simulink model "ads5296_snap2"  (R2019a)
settings: Solver=FixedStepAuto  StartTime=0.0  StopTime=10.0  RelTol=1e-3
libraries: xbsIndex_r4 x3026, casper_library_misc x9, xps_library x1
(part 1 of 30)
settings Model: Creator=jackh  LastModifiedBy=jackh
settings DataIOCC: ReturnWorkspaceOutputs=off
settings DebuggingCC: PregeneratedLibrarySubsystemCodeDiagnostic=none  ArithmeticOperatorsInVariantConditions=warning
settings SFSimCC: SimUseLocalCustomCode=off
settings RTWCC: RTWUseLocalCustomCode=off

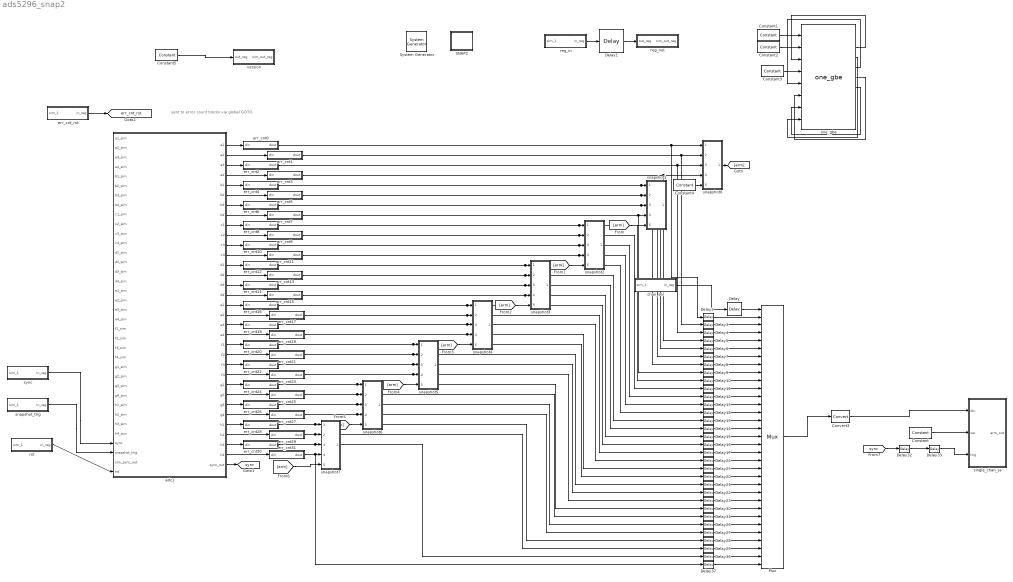
== system ads5296_snap2 ==
  note: sent to error count blocks via global GOTO.
  " System Generator" : xbsIndex_r4/ System Generator  Tag=genX  xilinxfamily=kintexu  part=xcku115  speed=-2-e  package=flvf1924  synthesis_tool=XST  clock_wrapper=Clock Enables  directory=/home/jackh/src/caltech-lwa/test_models/ads5296_snap2_clkswitch_c/sysgen  proj_type=Vivado  Synth_file=Vivado Synthesis Defaults  Impl_file=Vivado Implementation Defaults  testbench=off  simulink_period=1  sysclk_period=5  dcm_input_clock_period=10  incr_netlist=off  trim_vbits=Everywhere in SubSystem  dbl_ovrd=According to Block Masks  core_generation=According to Block Masks  run_coregen=off  deprecated_control=off  eval_field=0  block_type=sysgen
  Constant : xbsIndex_r4/Constant  const=1  gui_display_data_type=Boolean  arith_type=Boolean  n_bits=16  bin_pt=14  preci_type=Single  exp_width=8  frac_width=24  explicit_period=on  period=1  equ=P=C  opselect=C  inp2=PCIN>>17  opr=+  inp1=P  carry=CIN  dbl_ovrd=off  block_type=constant
  Constant{1..4} (4 alike) : xbsIndex_r4/Constant  const=0  gui_display_data_type=Boolean  arith_type=Boolean  n_bits=16  bin_pt=14  preci_type=Single  exp_width=8  frac_width=24  explicit_period=on  period=1  equ=P=C  opselect=C  inp2=PCIN>>17  opr=+  inp1=P  carry=CIN  dbl_ovrd=off  block_type=constant
  Constant5 : xbsIndex_r4/Constant  const=1  gui_display_data_type=Fixed-point  arith_type=Unsigned  n_bits=32  bin_pt=0  preci_type=Single  exp_width=8  frac_width=24  explicit_period=on  period=1  equ=P=C  opselect=C  inp2=PCIN>>17  opr=+  inp1=P  carry=CIN  dbl_ovrd=off  block_type=constant
  Convert3 : xbsIndex_r4/Convert  gui_display_data_type=Fixed-point  arith_type="Signed  (2's comp)"  n_bits=16  bin_pt=15  float_type=Single  exp_bits=8  fraction_bits=24  quantization=Truncate  overflow=Wrap  en=off  latency=0  pipeline=off  dbl_ovrd=off  block_type=convert
  Delay : xbsIndex_r4/Delay  rst=off  infoeditControl=Selection of Reset will increase slice count due to use of real FFs and instead of SRLs  en=off  latency=6  reg_retiming=on  dbl_ovrd=off  block_type=delay
  Delay1 : xbsIndex_r4/Delay  rst=off  infoeditControl=Selection of Reset will increase slice count due to use of real FFs and instead of SRLs  en=off  latency=1  reg_retiming=off  dbl_ovrd=off  block_type=delay
  Delay{2..32,36..37} (33 alike) : xbsIndex_r4/Delay  rst=off  infoeditControl=Selection of Reset will increase slice count due to use of real FFs and instead of SRLs  en=off  latency=2  reg_retiming=on  dbl_ovrd=off  block_type=delay
  Delay33 : xbsIndex_r4/Delay  rst=off  infoeditControl=Selection of Reset will increase slice count due to use of real FFs and instead of SRLs  en=off  latency=4  reg_retiming=on  dbl_ovrd=off  block_type=delay
  Mux : xbsIndex_r4/Mux  inputs=32  en=off  latency=4  precision=Full  arith_type=Unsigned  n_bits=16  bin_pt=14  quantization=Truncate  overflow=Wrap  dbl_ovrd=off  block_type=mux
  SNAP2 : Subsystem  Tag=xps:xsg  mask(xsg core config){hw_sys=SNAP2_v2:xcku115, clk_src=adc1_clk, clk_rate=200, use_microblaze=on, sample_period=1, synthesis_tool=XST}
      mask prompts: hw_sys "Hardware Platform"; clk_src "User IP Clock source"; clk_rate "User IP Clock Rate (MHz)"; use_microblaze "Use Microblaze controller?"; sample_period "Sample Period"; synthesis_tool "Synthesis Tool:"
      mask help:
      | The XSG Core Config block is used to configure the System Generator design
      | for the casper_xps toolflow. Settings here are used to configure the
      | Xilinx System Generator block parameters automatically, and control toolflow
      | script  execution. It needs to be at the top level of all designs being compiled
      | with the casper_xps toolflow.
      mask init:
      | xps_xsg_snap2_conf_mask;
      mask Help: eval('xlWeb([getenv(''MLIB_ROOT''), ''\doc\html\sys_xsg_core_config\sys_xsg_core_config.html''])')
      mask TypeOptions hw_sys: SNAP2_v1:xcku115 | SNAP2_v2:xcku115
      mask TypeOptions clk_src: sys_clk | clk_250MHz | adc0_clk | adc1_clk
      mask TypeOptions synthesis_tool: Leonardo Spectrum | Synplify | Synplify Pro | XST
      mask Display: fprintf(['SNAP2']);
  adc1 : Subsystem  Tag=xps:ads5296x4  mask(ADS5296x4){board_count=2, sample_rate=200, port=1, clockport=1, version=1}
      mask prompts: board_count "Number of quad-chip ADC Boards"; sample_rate "Sample Rate"; port "Which FMC port?"; clockport "Use clock from which FMC board?"; version "Which ADC board version?"
      mask help: 16-input ADC based on the TI ADS5296 chip.
      mask init:
      | % Only board_count is needed by init function
      | ads5296x4_init(gcb, ...
      |     'board_count', board_count);
      mask TypeOptions board_count: 1 | 2 | 3 | 4
  chan_sel : Subsystem  Tag=xps:sw_reg  AncestorBlock=xps_library/Memory/software_register  mask(swreg){io_dir=From Processor, io_delay=0, init_val=0, sample_period=1, names=reg, bitwidths=5, bin_pts=0, arith_types=0, sim_port=on, show_format=on}
      mask prompts: io_dir "I/O direction"; io_delay "I/O delay"; init_val "Initial Value"; sample_period "Sample period"; names "Bitfield names [msb...lsb]"; bitwidths "Bitfield widths"; bin_pts "Bitfield binary pts"; arith_types "Bitfield types, ufix=0, fix=1, bool=2"; sim_port "Provide sim input/output?"; show_format "Print format string?"
      mask help: A 32-bit software-accessible register. Can be divided into bitfields of varying widths and types using the fields in the block mask.
      mask init:
      | swreg_init(gcb)
      settings: AttributesFormatString=1input:uf5.0 = 5 bits
      mask TypeOptions io_dir: To Processor | From Processor
      mask Callback io_dir:
      | mask_enables = get_param(gcb, 'MaskEnables');
      | mask_names = get_param(gcb, 'MaskNames');
      | if strcmp(get_param(gcb, 'io_dir'), 'To Processor'),
      |     mask_enables{ismember(mask_names, 'sample_period')} = 'off';
      | else
      |     mask_enables{ismember(mask_names, 'sample_period')} = 'on';
      | end
      | set_param(gcb, 'MaskEnables', mask_enables);
      mask DialogControl ParameterTabVar0 Prompt: Setup
  err_cnt0 : Subsystem  VariantControl=Variant1
  err_cnt1 : Subsystem  VariantControl=Variant1
  err_cnt10 : Subsystem  VariantControl=Variant1
  err_cnt11 : Subsystem  VariantControl=Variant1
  err_cnt12 : Subsystem  VariantControl=Variant1
  err_cnt13 : Subsystem  VariantControl=Variant1
  err_cnt14 : Subsystem  VariantControl=Variant1
  err_cnt15 : Subsystem  VariantControl=Variant1
  err_cnt16 : Subsystem  VariantControl=Variant1
  err_cnt17 : Subsystem  VariantControl=Variant1
  err_cnt18 : Subsystem  VariantControl=Variant1
  err_cnt19 : Subsystem  VariantControl=Variant1
  err_cnt2 : Subsystem  VariantControl=Variant1
  err_cnt20 : Subsystem  VariantControl=Variant1
  err_cnt21 : Subsystem  VariantControl=Variant1
  err_cnt22 : Subsystem  VariantControl=Variant1
  err_cnt23 : Subsystem  VariantControl=Variant1
  err_cnt24 : Subsystem  VariantControl=Variant1
  err_cnt25 : Subsystem  VariantControl=Variant1
  err_cnt26 : Subsystem  VariantControl=Variant1
  err_cnt27 : Subsystem  VariantControl=Variant1
  err_cnt28 : Subsystem  VariantControl=Variant1
  err_cnt29 : Subsystem  VariantControl=Variant1
  err_cnt3 : Subsystem  VariantControl=Variant1
  err_cnt30 : Subsystem  VariantControl=Variant1
  err_cnt31 : Subsystem  VariantControl=Variant1
  err_cnt4 : Subsystem  VariantControl=Variant1
  err_cnt5 : Subsystem  VariantControl=Variant1
  err_cnt6 : Subsystem  VariantControl=Variant1
  err_cnt7 : Subsystem  VariantControl=Variant1
  err_cnt8 : Subsystem  VariantControl=Variant1
  err_cnt9 : Subsystem  VariantControl=Variant1
  err_cnt_rst : Subsystem  Tag=xps:sw_reg  AncestorBlock=xps_library/Memory/software_register  mask(swreg){io_dir=From Processor, io_delay=0, init_val=0, sample_period=1, names=reg, bitwidths=1, bin_pts=0, arith_types=2, sim_port=on, show_format=on}
      mask prompts: io_dir "I/O direction"; io_delay "I/O delay"; init_val "Initial Value"; sample_period "Sample period"; names "Bitfield names [msb...lsb]"; bitwidths "Bitfield widths"; bin_pts "Bitfield binary pts"; arith_types "Bitfield types, ufix=0, fix=1, bool=2"; sim_port "Provide sim input/output?"; show_format "Print format string?"
      mask help: A 32-bit software-accessible register. Can be divided into bitfields of varying widths and types using the fields in the block mask.
      mask init:
      | swreg_init(gcb)
      settings: AttributesFormatString=1input:b = 1 bits
      mask TypeOptions io_dir: To Processor | From Processor
      mask Callback io_dir:
      | mask_enables = get_param(gcb, 'MaskEnables');
      | mask_names = get_param(gcb, 'MaskNames');
      | if strcmp(get_param(gcb, 'io_dir'), 'To Processor'),
      |     mask_enables{ismember(mask_names, 'sample_period')} = 'off';
      | else
      |     mask_enables{ismember(mask_names, 'sample_period')} = 'on';
      | end
      | set_param(gcb, 'MaskEnables', mask_enables);
      mask DialogControl ParameterTabVar0 Prompt: Setup
  one_gbe : xps_library/IO/one_gbe  Tag=xps:onegbe  local_en=on  dis_cpu_rx=off  dis_cpu_tx=off  cpu_promiscuous=on  local_mac=hex2dec('123456789abc')  local_ip=hex2dec('c0a8290a')  local_port=4321  local_gateway=1
      settings: SourceProductName=CASPER XPS Blockset
  reg_in : Subsystem  Tag=xps:sw_reg  AncestorBlock=xps_library/Memory/software_register  mask(swreg){io_dir=From Processor, io_delay=0, init_val=0, sample_period=1, names=reg, bitwidths=10, bin_pts=9, arith_types=1, sim_port=on, show_format=on}
      mask prompts: io_dir "I/O direction"; io_delay "I/O delay"; init_val "Initial Value"; sample_period "Sample period"; names "Bitfield names [msb...lsb]"; bitwidths "Bitfield widths"; bin_pts "Bitfield binary pts"; arith_types "Bitfield types, ufix=0, fix=1, bool=2"; sim_port "Provide sim input/output?"; show_format "Print format string?"
      mask help: A 32-bit software-accessible register. Can be divided into bitfields of varying widths and types using the fields in the block mask.
      mask init:
      | swreg_init(gcb)
      settings: AttributesFormatString=1input:f10.9 = 10 bits
      mask TypeOptions io_dir: To Processor | From Processor
      mask Callback io_dir:
      | mask_enables = get_param(gcb, 'MaskEnables');
      | mask_names = get_param(gcb, 'MaskNames');
      | if strcmp(get_param(gcb, 'io_dir'), 'To Processor'),
      |     mask_enables{ismember(mask_names, 'sample_period')} = 'off';
      | else
      |     mask_enables{ismember(mask_names, 'sample_period')} = 'on';
      | end
      | set_param(gcb, 'MaskEnables', mask_enables);
      mask DialogControl ParameterTabVar0 Prompt: Setup
  reg_out : Subsystem  Tag=xps:sw_reg  AncestorBlock=xps_library/Memory/software_register  mask(swreg){io_dir=To Processor, io_delay=0, init_val=0, sample_period=1, names=reg, bitwidths=10, bin_pts=9, arith_types=1, sim_port=on, show_format=on}
      mask prompts: io_dir "I/O direction"; io_delay "I/O delay"; init_val "Initial Value"; sample_period "Sample period"; names "Bitfield names [msb...lsb]"; bitwidths "Bitfield widths"; bin_pts "Bitfield binary pts"; arith_types "Bitfield types, ufix=0, fix=1, bool=2"; sim_port "Provide sim input/output?"; show_format "Print format string?"
      mask help: A 32-bit software-accessible register. Can be divided into bitfields of varying widths and types using the fields in the block mask.
      mask init:
      | swreg_init(gcb)
      settings: AttributesFormatString=1output:f10.9 = 10 bits
      mask TypeOptions io_dir: To Processor | From Processor
      mask Callback io_dir:
      | mask_enables = get_param(gcb, 'MaskEnables');
      | mask_names = get_param(gcb, 'MaskNames');
      | if strcmp(get_param(gcb, 'io_dir'), 'To Processor'),
      |     mask_enables{ismember(mask_names, 'sample_period')} = 'off';
      | else
      |     mask_enables{ismember(mask_names, 'sample_period')} = 'on';
      | end
      | set_param(gcb, 'MaskEnables', mask_enables);
      mask DialogControl ParameterTabVar0 Prompt: Setup
  rst : Subsystem  Tag=xps:sw_reg  AncestorBlock=xps_library/Memory/software_register  mask(swreg){io_dir=From Processor, io_delay=0, init_val=0, sample_period=1, names=reg, bitwidths=1, bin_pts=0, arith_types=2, sim_port=on, show_format=on}
      mask prompts: io_dir "I/O direction"; io_delay "I/O delay"; init_val "Initial Value"; sample_period "Sample period"; names "Bitfield names [msb...lsb]"; bitwidths "Bitfield widths"; bin_pts "Bitfield binary pts"; arith_types "Bitfield types, ufix=0, fix=1, bool=2"; sim_port "Provide sim input/output?"; show_format "Print format string?"
      mask help: A 32-bit software-accessible register. Can be divided into bitfields of varying widths and types using the fields in the block mask.
      mask init:
      | swreg_init(gcb)
      settings: AttributesFormatString=1input:b = 1 bits
      mask TypeOptions io_dir: To Processor | From Processor
      mask Callback io_dir:
      | mask_enables = get_param(gcb, 'MaskEnables');
      | mask_names = get_param(gcb, 'MaskNames');
      | if strcmp(get_param(gcb, 'io_dir'), 'To Processor'),
      |     mask_enables{ismember(mask_names, 'sample_period')} = 'off';
      | else
      |     mask_enables{ismember(mask_names, 'sample_period')} = 'on';
      | end
      | set_param(gcb, 'MaskEnables', mask_enables);
      mask DialogControl ParameterTabVar0 Prompt: Setup
  single_chan_ss : Subsystem  Tag=casper:snapshot  AncestorBlock=casper_library_scopes/snapshot  mask(snapshot){storage=bram, dram_dimm=2, dram_clock=250, nsamples=16, data_width=16, offset=off, circap=off, value=off, ext_arm=off, ext_circ=off, provide_outputs=on, use_dsp48=off}
      mask prompts: storage "Storage medium"; dram_dimm "DRAM dimm"; dram_clock "DRAM clock rate"; nsamples "Number of Samples (2^?)"; data_width "Data width"; offset "Start delay support"; circap "Circular capture support"; value "Extra value capture support"; ext_arm "External arm support"; ext_circ "External circular capture support"; provide_outputs "Provide outputs"; use_dsp48 "Use DSP48s to implement counters"
      mask help:
      | Standard snap block, but with the following optional extras;
      |  1) Optionally delay the fabric trigger by a user-specified number of valids.
      |  2) Capture continuously after a trigger until a stop pulse is received. Data is captured into BRAM continuously, with old data being overwritten until a stop command is received. Then stop capturing when memory is filled. This enables you to get some data before and some data after the stop pulse. Use the 'tr_en_cnt' register to determine where you are in your vector. 'Addr' register's MSb now indicates 'busy capturing'.
      |  3) Optionally capture a value on an input port to a register at the same time as the first data sample.
      |  4) Implement counters using DSP48Es to save resources.
      mask init:
      | snapshot_init(gcb, ...
      |     'storage', storage, ...
      |     'dram_dimm', dram_dimm, ...
      |     'dram_clock', dram_clock, ...
      |     'nsamples', nsamples, ...
      |     'data_width', data_width, ...
      |     'offset', offset, ...
      |     'circap', circap, ...
      |     'value', value, ...
      |     'ext_arm', ext_arm, ...
      |     'ext_circ', ext_circ, ...
      |     'provide_outputs', 'off', ...
      |     'use_dsp48', use_dsp48);
      settings: AttributesFormatString=|
      | 16 wide, 65536 deep
      | debugID: 35264124
      mask TypeOptions storage: bram | dram
      mask Callback storage: snapshot_callback();
      mask TypeOptions dram_dimm: 1 | 2 | 3 | 4
      mask TypeOptions dram_clock: 200 | 250 | 266 | 300 | 333
      mask TypeOptions data_width: 8 | 16 | 32 | 64 | 128
  snapshot0 : Subsystem
  snapshot1 : Subsystem
  snapshot2 : Subsystem
  snapshot3 : Subsystem
  snapshot4 : Subsystem
  snapshot5 : Subsystem
  snapshot6 : Subsystem
  snapshot7 : Subsystem
  snapshot_trig : Subsystem  Tag=xps:sw_reg  AncestorBlock=xps_library/Memory/software_register  mask(swreg){io_dir=From Processor, io_delay=0, init_val=0, sample_period=1, names=reg, bitwidths=1, bin_pts=0, arith_types=2, sim_port=on, show_format=on}
      mask prompts: io_dir "I/O direction"; io_delay "I/O delay"; init_val "Initial Value"; sample_period "Sample period"; names "Bitfield names [msb...lsb]"; bitwidths "Bitfield widths"; bin_pts "Bitfield binary pts"; arith_types "Bitfield types, ufix=0, fix=1, bool=2"; sim_port "Provide sim input/output?"; show_format "Print format string?"
      mask help: A 32-bit software-accessible register. Can be divided into bitfields of varying widths and types using the fields in the block mask.
      mask init:
      | swreg_init(gcb)
      settings: AttributesFormatString=1input:b = 1 bits
      mask TypeOptions io_dir: To Processor | From Processor
      mask Callback io_dir:
      | mask_enables = get_param(gcb, 'MaskEnables');
      | mask_names = get_param(gcb, 'MaskNames');
      | if strcmp(get_param(gcb, 'io_dir'), 'To Processor'),
      |     mask_enables{ismember(mask_names, 'sample_period')} = 'off';
      | else
      |     mask_enables{ismember(mask_names, 'sample_period')} = 'on';
      | end
      | set_param(gcb, 'MaskEnables', mask_enables);
      mask DialogControl ParameterTabVar0 Prompt: Setup
  sync : Subsystem  Tag=xps:sw_reg  AncestorBlock=xps_library/Memory/software_register  mask(swreg){io_dir=From Processor, io_delay=0, init_val=0, sample_period=1, names=reg, bitwidths=1, bin_pts=0, arith_types=2, sim_port=on, show_format=on}
      mask prompts: io_dir "I/O direction"; io_delay "I/O delay"; init_val "Initial Value"; sample_period "Sample period"; names "Bitfield names [msb...lsb]"; bitwidths "Bitfield widths"; bin_pts "Bitfield binary pts"; arith_types "Bitfield types, ufix=0, fix=1, bool=2"; sim_port "Provide sim input/output?"; show_format "Print format string?"
      mask help: A 32-bit software-accessible register. Can be divided into bitfields of varying widths and types using the fields in the block mask.
      mask init:
      | swreg_init(gcb)
      settings: AttributesFormatString=1input:b = 1 bits
      mask TypeOptions io_dir: To Processor | From Processor
      mask Callback io_dir:
      | mask_enables = get_param(gcb, 'MaskEnables');
      | mask_names = get_param(gcb, 'MaskNames');
      | if strcmp(get_param(gcb, 'io_dir'), 'To Processor'),
      |     mask_enables{ismember(mask_names, 'sample_period')} = 'off';
      | else
      |     mask_enables{ismember(mask_names, 'sample_period')} = 'on';
      | end
      | set_param(gcb, 'MaskEnables', mask_enables);
      mask DialogControl ParameterTabVar0 Prompt: Setup
  version : Subsystem  Tag=xps:sw_reg  AncestorBlock=xps_library/Memory/software_register  mask(swreg){io_dir=To Processor, io_delay=0, init_val=0, sample_period=1, names=reg, bitwidths=32, bin_pts=0, arith_types=0, sim_port=on, show_format=on}
      mask prompts: io_dir "I/O direction"; io_delay "I/O delay"; init_val "Initial Value"; sample_period "Sample period"; names "Bitfield names [msb...lsb]"; bitwidths "Bitfield widths"; bin_pts "Bitfield binary pts"; arith_types "Bitfield types, ufix=0, fix=1, bool=2"; sim_port "Provide sim input/output?"; show_format "Print format string?"
      mask help: A 32-bit software-accessible register. Can be divided into bitfields of varying widths and types using the fields in the block mask.
      mask init:
      | swreg_init(gcb)
      settings: AttributesFormatString=1output:uf32.0 = 32 bits
      mask TypeOptions io_dir: To Processor | From Processor
      mask Callback io_dir:
      | mask_enables = get_param(gcb, 'MaskEnables');
      | mask_names = get_param(gcb, 'MaskNames');
      | if strcmp(get_param(gcb, 'io_dir'), 'To Processor'),
      |     mask_enables{ismember(mask_names, 'sample_period')} = 'off';
      | else
      |     mask_enables{ismember(mask_names, 'sample_period')} = 'on';
      | end
      | set_param(gcb, 'MaskEnables', mask_enables);
      mask DialogControl ParameterTabVar0 Prompt: Setup
  tag scope: err_cnt_rst=global, sync=global
  wires:
  reg_in/1(in_reg) -> Delay1/1
  Delay1/1 -> reg_out/1(out_reg)
  sync/1(in_reg) -> adc1/33(sync)
  rst/1(in_reg) -> adc1/36(rst)
  adc1/4(a4) -> err_cnt3/1(din)
  adc1/3(a3) -> err_cnt2/1(din)
  adc1/2(a2) -> err_cnt1/1(din)
  Constant1/1 -> one_gbe/1
  Constant2/1 -> one_gbe/2
  one_gbe/3 -> one_gbe/3
  Constant3/1 -> one_gbe/4
  one_gbe/5 -> one_gbe/5
  one_gbe/6 -> one_gbe/6
  one_gbe/7 -> one_gbe/7
  one_gbe/4 -> one_gbe/8
  Constant4/1 -> snapshot0/5(arm_in)
  [arm] -> snapshot1/5(arm_in)
  snapshot0/1(arm) -> [arm]
  adc1/5(b1) -> err_cnt4/1(din)
  adc1/6(b2) -> err_cnt5/1(din)
  adc1/7(b3) -> err_cnt6/1(din)
  adc1/8(b4) -> err_cnt7/1(din)
  adc1/12(c4) -> err_cnt11/1(din)
  adc1/11(c3) -> err_cnt10/1(din)
  adc1/10(c2) -> err_cnt9/1(din)
  adc1/9(c1) -> err_cnt8/1(din)
  [arm] -> snapshot2/5(arm_in)
  [arm] -> snapshot3/5(arm_in)
  adc1/13(d1) -> err_cnt12/1(din)
  adc1/14(d2) -> err_cnt13/1(din)
  adc1/15(d3) -> err_cnt14/1(din)
  adc1/16(d4) -> err_cnt15/1(din)
  [arm] -> snapshot4/5(arm_in)
  adc1/17(e1) -> err_cnt16/1(din)
  adc1/18(e2) -> err_cnt17/1(din)
  [arm] -> snapshot5/5(arm_in)
  [arm] -> snapshot6/5(arm_in)
  adc1/21(f1) -> err_cnt20/1(din)
  adc1/23(f3) -> err_cnt22/1(din)
  adc1/25(g1) -> err_cnt24/1(din)
  adc1/27(g3) -> err_cnt26/1(din)
  [arm] -> snapshot7/5(arm_in)
  adc1/29(h1) -> err_cnt28/1(din)
  adc1/30(h2) -> err_cnt29/1(din)
  adc1/31(h3) -> err_cnt30/1(din)
  adc1/32(h4) -> err_cnt31/1(din)
  adc1/33(sync_out) -> [sync]
  chan_sel/1(in_reg) -> Delay/1
  Delay/1 -> Mux/1
  Delay2/1 -> Mux/2
  Delay3/1 -> Mux/3
  Delay4/1 -> Mux/4
  Delay5/1 -> Mux/5
  Delay6/1 -> Mux/6
  Delay7/1 -> Mux/7
  Delay8/1 -> Mux/8
  Delay13/1 -> Mux/13
  Delay9/1 -> Mux/9
  Delay12/1 -> Mux/12
  Delay10/1 -> Mux/10
  Delay11/1 -> Mux/11
  Delay19/1 -> Mux/15
  Delay17/1 -> Mux/19
  Delay14/1 -> Mux/16
  Delay16/1 -> Mux/18
  Delay18/1 -> Mux/14
  Delay15/1 -> Mux/17
  Delay20/1 -> Mux/22
  Delay23/1 -> Mux/25
  Delay24/1 -> Mux/20
  Delay25/1 -> Mux/21
  Delay21/1 -> Mux/23
  Delay22/1 -> Mux/24
  Delay27/1 -> Mux/29
  Delay30/1 -> Mux/26
  Delay29/1 -> Mux/31
  Delay31/1 -> Mux/27
  Delay26/1 -> Mux/28
  Delay28/1 -> Mux/30
  Delay37/1 -> Mux/33
  Delay36/1 -> Mux/32
  [sync] -> Delay32/1
  Constant/1 -> single_chan_ss/2(we)
  Convert3/1 -> single_chan_ss/1(din)
  Mux/1 -> Convert3/1
  Delay32/1 -> Delay33/1
  Delay33/1 -> single_chan_ss/3(trig)
  err_cnt_rst/1(in_reg) -> [err_cnt_rst]
  err_cnt1/1(dout) -> snapshot0/2(din1), Delay3/1
  err_cnt2/1(dout) -> Delay4/1, snapshot0/3(din2)
  err_cnt3/1(dout) -> Delay5/1, snapshot0/4(din3)
  err_cnt5/1(dout) -> snapshot1/2(din1), Delay7/1
  err_cnt7/1(dout) -> Delay9/1, snapshot1/4(din3)
  err_cnt4/1(dout) -> snapshot1/1(din0), Delay6/1
  err_cnt6/1(dout) -> snapshot1/3(din2), Delay8/1
  err_cnt13/1(dout) -> Delay19/1, snapshot3/2(din1)
  err_cnt8/1(dout) -> Delay10/1, snapshot2/1(din0)
  err_cnt9/1(dout) -> snapshot2/2(din1), Delay11/1
  err_cnt14/1(dout) -> Delay14/1, snapshot3/3(din2)
  err_cnt15/1(dout) -> snapshot3/4(din3), Delay15/1
  err_cnt10/1(dout) -> snapshot2/3(din2), Delay12/1
  err_cnt11/1(dout) -> snapshot2/4(din3), Delay13/1
  err_cnt12/1(dout) -> snapshot3/1(din0), Delay18/1
  adc1/19(e3) -> err_cnt18/1(din)
  err_cnt22/1(dout) -> snapshot5/3(din2), Delay22/1
  adc1/22(f2) -> err_cnt21/1(din)
  adc1/24(f4) -> err_cnt23/1(din)
  err_cnt16/1(dout) -> snapshot4/1(din0), Delay16/1
  err_cnt20/1(dout) -> Delay20/1, snapshot5/1(din0)
  adc1/20(e4) -> err_cnt19/1(din)
  err_cnt17/1(dout) -> snapshot4/2(din1), Delay17/1
  err_cnt26/1(dout) -> snapshot6/3(din2), Delay26/1
  adc1/28(g4) -> err_cnt27/1(din)
  err_cnt28/1(dout) -> Delay28/1, snapshot7/1(din0)
  err_cnt29/1(dout) -> snapshot7/2(din1), Delay29/1
  err_cnt30/1(dout) -> snapshot7/3(din2), Delay36/1
  err_cnt31/1(dout) -> Delay37/1, snapshot7/4(din3)
  err_cnt24/1(dout) -> Delay30/1, snapshot6/1(din0)
  adc1/26(g2) -> err_cnt25/1(din)
  err_cnt18/1(dout) -> snapshot4/3(din2), Delay24/1
  err_cnt19/1(dout) -> Delay25/1, snapshot4/4(din3)
  err_cnt21/1(dout) -> snapshot5/2(din1), Delay21/1
  err_cnt23/1(dout) -> snapshot5/4(din3), Delay23/1
  err_cnt25/1(dout) -> Delay31/1, snapshot6/2(din1)
  err_cnt27/1(dout) -> snapshot6/4(din3), Delay27/1
  adc1/1(a1) -> err_cnt0/1(din)
  err_cnt0/1(dout) -> snapshot0/1(din0), Delay2/1
  snapshot_trig/1(in_reg) -> adc1/34(snapshot_trig)
  Constant5/1 -> version/1(out_reg)

== system ads5296_snap2/SNAP2 ==

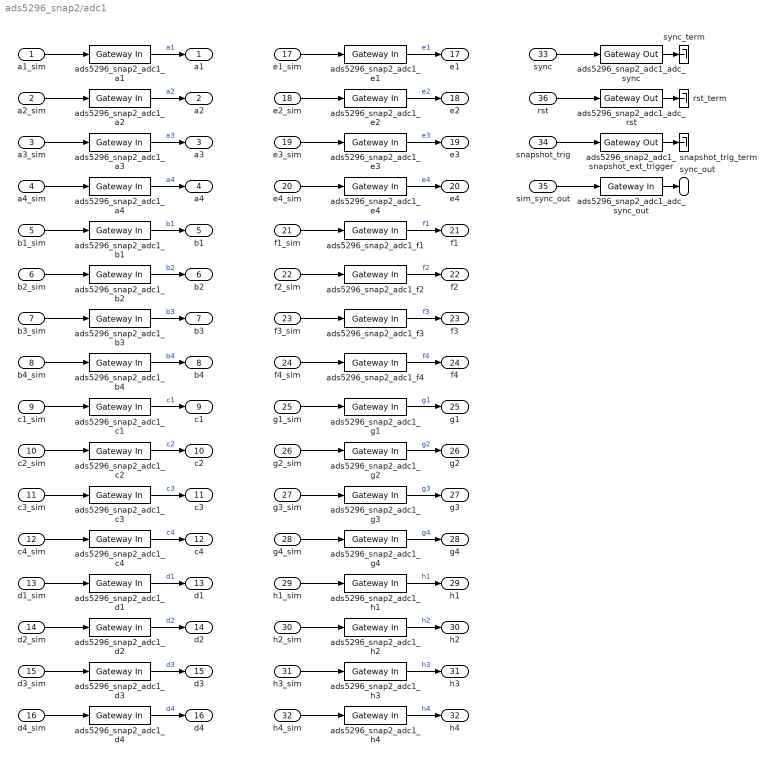
== system ads5296_snap2/adc1 ==
  a1_sim : Inport
  a2_sim : Inport  Port=2
  a3_sim : Inport  Port=3
  a4_sim : Inport  Port=4
  b1_sim : Inport  Port=5
  b2_sim : Inport  Port=6
  b3_sim : Inport  Port=7
  b4_sim : Inport  Port=8
  c1_sim : Inport  Port=9
  c2_sim : Inport  Port=10
  c3_sim : Inport  Port=11
  c4_sim : Inport  Port=12
  d1_sim : Inport  Port=13
  d2_sim : Inport  Port=14
  d3_sim : Inport  Port=15
  d4_sim : Inport  Port=16
  e1_sim : Inport  Port=17
  e2_sim : Inport  Port=18
  e3_sim : Inport  Port=19
  e4_sim : Inport  Port=20
  f1_sim : Inport  Port=21
  f2_sim : Inport  Port=22
  f3_sim : Inport  Port=23
  f4_sim : Inport  Port=24
  g1_sim : Inport  Port=25
  g2_sim : Inport  Port=26
  g3_sim : Inport  Port=27
  g4_sim : Inport  Port=28
  h1_sim : Inport  Port=29
  h2_sim : Inport  Port=30
  h3_sim : Inport  Port=31
  h4_sim : Inport  Port=32
  sync : Inport  Port=33
  snapshot_trig : Inport  Port=34
  sim_sync_out : Inport  Port=35
  rst : Inport  Port=36
  ads5296_snap2_adc1_a{1..4} (4 alike) : xbsIndex_r4/Gateway In  gui_display_data_type=Fixed-point  arith_type="Signed  (2's comp)"  n_bits=10  bin_pt=9  preci_type=Single  exp_width=8  frac_width=24  rows=1  columns=1  quantization="Round  (unbiased: +/- Inf)"  overflow=Saturate  period=1  UseAsADC=off  ADCChannel='1'  interface=None  automatic_assignment=on  address_offset=hex2dec('00')  intf_name=''  intf_description=''  default_value=0  timing_constraint=None  locs_specified=off  LOCs={}  io_standard={}  inherit_from_input=off  hdl_port=on  dbl_ovrd=off  block_type=gatewayin
  ads5296_snap2_adc1_adc_rst : xbsIndex_r4/Gateway Out  inherit_from_input=off  hdl_port=on  rows=1  columns=1  UseAsDAC=off  DACChannel='1'  interface=None  automatic_assignment=on  address_offset=hex2dec('00')  intf_name=''  intf_description=''  timing_constraint=None  locs_specified=off  LOCs={}  io_standard={}  block_type=gatewayout
  ads5296_snap2_adc1_adc_sync : xbsIndex_r4/Gateway Out  inherit_from_input=off  hdl_port=on  rows=1  columns=1  UseAsDAC=off  DACChannel='1'  interface=None  automatic_assignment=on  address_offset=hex2dec('00')  intf_name=''  intf_description=''  timing_constraint=None  locs_specified=off  LOCs={}  io_standard={}  block_type=gatewayout
  ads5296_snap2_adc1_adc_sync_out : xbsIndex_r4/Gateway In  gui_display_data_type=Fixed-point  arith_type=Boolean  n_bits=16  bin_pt=14  preci_type=Single  exp_width=8  frac_width=24  rows=1  columns=1  quantization="Round  (unbiased: +/- Inf)"  overflow=Saturate  period=1  UseAsADC=off  ADCChannel='1'  interface=None  automatic_assignment=on  address_offset=hex2dec('00')  intf_name=''  intf_description=''  default_value=0  timing_constraint=None  locs_specified=off  LOCs={}  io_standard={}  inherit_from_input=off  hdl_port=on  dbl_ovrd=off  block_type=gatewayin
  ads5296_snap2_adc1_b{1..4} (4 alike) : xbsIndex_r4/Gateway In  gui_display_data_type=Fixed-point  arith_type="Signed  (2's comp)"  n_bits=10  bin_pt=9  preci_type=Single  exp_width=8  frac_width=24  rows=1  columns=1  quantization="Round  (unbiased: +/- Inf)"  overflow=Saturate  period=1  UseAsADC=off  ADCChannel='1'  interface=None  automatic_assignment=on  address_offset=hex2dec('00')  intf_name=''  intf_description=''  default_value=0  timing_constraint=None  locs_specified=off  LOCs={}  io_standard={}  inherit_from_input=off  hdl_port=on  dbl_ovrd=off  block_type=gatewayin
  ads5296_snap2_adc1_c{1..4} (4 alike) : xbsIndex_r4/Gateway In  gui_display_data_type=Fixed-point  arith_type="Signed  (2's comp)"  n_bits=10  bin_pt=9  preci_type=Single  exp_width=8  frac_width=24  rows=1  columns=1  quantization="Round  (unbiased: +/- Inf)"  overflow=Saturate  period=1  UseAsADC=off  ADCChannel='1'  interface=None  automatic_assignment=on  address_offset=hex2dec('00')  intf_name=''  intf_description=''  default_value=0  timing_constraint=None  locs_specified=off  LOCs={}  io_standard={}  inherit_from_input=off  hdl_port=on  dbl_ovrd=off  block_type=gatewayin
  ads5296_snap2_adc1_d{1..4} (4 alike) : xbsIndex_r4/Gateway In  gui_display_data_type=Fixed-point  arith_type="Signed  (2's comp)"  n_bits=10  bin_pt=9  preci_type=Single  exp_width=8  frac_width=24  rows=1  columns=1  quantization="Round  (unbiased: +/- Inf)"  overflow=Saturate  period=1  UseAsADC=off  ADCChannel='1'  interface=None  automatic_assignment=on  address_offset=hex2dec('00')  intf_name=''  intf_description=''  default_value=0  timing_constraint=None  locs_specified=off  LOCs={}  io_standard={}  inherit_from_input=off  hdl_port=on  dbl_ovrd=off  block_type=gatewayin
  ads5296_snap2_adc1_e{1..4} (4 alike) : xbsIndex_r4/Gateway In  gui_display_data_type=Fixed-point  arith_type="Signed  (2's comp)"  n_bits=10  bin_pt=9  preci_type=Single  exp_width=8  frac_width=24  rows=1  columns=1  quantization="Round  (unbiased: +/- Inf)"  overflow=Saturate  period=1  UseAsADC=off  ADCChannel='1'  interface=None  automatic_assignment=on  address_offset=hex2dec('00')  intf_name=''  intf_description=''  default_value=0  timing_constraint=None  locs_specified=off  LOCs={}  io_standard={}  inherit_from_input=off  hdl_port=on  dbl_ovrd=off  block_type=gatewayin
  ads5296_snap2_adc1_f{1..4} (4 alike) : xbsIndex_r4/Gateway In  gui_display_data_type=Fixed-point  arith_type="Signed  (2's comp)"  n_bits=10  bin_pt=9  preci_type=Single  exp_width=8  frac_width=24  rows=1  columns=1  quantization="Round  (unbiased: +/- Inf)"  overflow=Saturate  period=1  UseAsADC=off  ADCChannel='1'  interface=None  automatic_assignment=on  address_offset=hex2dec('00')  intf_name=''  intf_description=''  default_value=0  timing_constraint=None  locs_specified=off  LOCs={}  io_standard={}  inherit_from_input=off  hdl_port=on  dbl_ovrd=off  block_type=gatewayin
  ads5296_snap2_adc1_g{1..4} (4 alike) : xbsIndex_r4/Gateway In  gui_display_data_type=Fixed-point  arith_type="Signed  (2's comp)"  n_bits=10  bin_pt=9  preci_type=Single  exp_width=8  frac_width=24  rows=1  columns=1  quantization="Round  (unbiased: +/- Inf)"  overflow=Saturate  period=1  UseAsADC=off  ADCChannel='1'  interface=None  automatic_assignment=on  address_offset=hex2dec('00')  intf_name=''  intf_description=''  default_value=0  timing_constraint=None  locs_specified=off  LOCs={}  io_standard={}  inherit_from_input=off  hdl_port=on  dbl_ovrd=off  block_type=gatewayin
  ads5296_snap2_adc1_h{1..4} (4 alike) : xbsIndex_r4/Gateway In  gui_display_data_type=Fixed-point  arith_type="Signed  (2's comp)"  n_bits=10  bin_pt=9  preci_type=Single  exp_width=8  frac_width=24  rows=1  columns=1  quantization="Round  (unbiased: +/- Inf)"  overflow=Saturate  period=1  UseAsADC=off  ADCChannel='1'  interface=None  automatic_assignment=on  address_offset=hex2dec('00')  intf_name=''  intf_description=''  default_value=0  timing_constraint=None  locs_specified=off  LOCs={}  io_standard={}  inherit_from_input=off  hdl_port=on  dbl_ovrd=off  block_type=gatewayin
  ads5296_snap2_adc1_snapshot_ext_trigger : xbsIndex_r4/Gateway Out  inherit_from_input=off  hdl_port=on  rows=1  columns=1  UseAsDAC=off  DACChannel='1'  interface=None  automatic_assignment=on  address_offset=hex2dec('00')  intf_name=''  intf_description=''  timing_constraint=None  locs_specified=off  LOCs={}  io_standard={}  block_type=gatewayout
  rst_term : Terminator
  snapshot_trig_term : Terminator
  sync_term : Terminator
  a1 : Outport
  a2 : Outport  Port=2
  a3 : Outport  Port=3
  a4 : Outport  Port=4
  b1 : Outport  Port=5
  b2 : Outport  Port=6
  b3 : Outport  Port=7
  b4 : Outport  Port=8
  c1 : Outport  Port=9
  c2 : Outport  Port=10
  c3 : Outport  Port=11
  c4 : Outport  Port=12
  d1 : Outport  Port=13
  d2 : Outport  Port=14
  d3 : Outport  Port=15
  d4 : Outport  Port=16
  e1 : Outport  Port=17
  e2 : Outport  Port=18
  e3 : Outport  Port=19
  e4 : Outport  Port=20
  f1 : Outport  Port=21
  f2 : Outport  Port=22
  f3 : Outport  Port=23
  f4 : Outport  Port=24
  g1 : Outport  Port=25
  g2 : Outport  Port=26
  g3 : Outport  Port=27
  g4 : Outport  Port=28
  h1 : Outport  Port=29
  h2 : Outport  Port=30
  h3 : Outport  Port=31
  h4 : Outport  Port=32
  sync_out : Outport  Port=33
  wires:
  a1_sim/1 -> ads5296_snap2_adc1_a1/1
  ads5296_snap2_adc1_a1/1 -> a1/1  "a1"
  a2_sim/1 -> ads5296_snap2_adc1_a2/1
  ads5296_snap2_adc1_a2/1 -> a2/1  "a2"
  a3_sim/1 -> ads5296_snap2_adc1_a3/1
  ads5296_snap2_adc1_a3/1 -> a3/1  "a3"
  a4_sim/1 -> ads5296_snap2_adc1_a4/1
  ads5296_snap2_adc1_a4/1 -> a4/1  "a4"
  b1_sim/1 -> ads5296_snap2_adc1_b1/1
  ads5296_snap2_adc1_b1/1 -> b1/1  "b1"
  b2_sim/1 -> ads5296_snap2_adc1_b2/1
  ads5296_snap2_adc1_b2/1 -> b2/1  "b2"
  b3_sim/1 -> ads5296_snap2_adc1_b3/1
  ads5296_snap2_adc1_b3/1 -> b3/1  "b3"
  b4_sim/1 -> ads5296_snap2_adc1_b4/1
  ads5296_snap2_adc1_b4/1 -> b4/1  "b4"
  c1_sim/1 -> ads5296_snap2_adc1_c1/1
  ads5296_snap2_adc1_c1/1 -> c1/1  "c1"
  c2_sim/1 -> ads5296_snap2_adc1_c2/1
  ads5296_snap2_adc1_c2/1 -> c2/1  "c2"
  c3_sim/1 -> ads5296_snap2_adc1_c3/1
  ads5296_snap2_adc1_c3/1 -> c3/1  "c3"
  c4_sim/1 -> ads5296_snap2_adc1_c4/1
  ads5296_snap2_adc1_c4/1 -> c4/1  "c4"
  d1_sim/1 -> ads5296_snap2_adc1_d1/1
  ads5296_snap2_adc1_d1/1 -> d1/1  "d1"
  d2_sim/1 -> ads5296_snap2_adc1_d2/1
  ads5296_snap2_adc1_d2/1 -> d2/1  "d2"
  d3_sim/1 -> ads5296_snap2_adc1_d3/1
  ads5296_snap2_adc1_d3/1 -> d3/1  "d3"
  d4_sim/1 -> ads5296_snap2_adc1_d4/1
  ads5296_snap2_adc1_d4/1 -> d4/1  "d4"
  e1_sim/1 -> ads5296_snap2_adc1_e1/1
  ads5296_snap2_adc1_e1/1 -> e1/1  "e1"
  e2_sim/1 -> ads5296_snap2_adc1_e2/1
  ads5296_snap2_adc1_e2/1 -> e2/1  "e2"
  e3_sim/1 -> ads5296_snap2_adc1_e3/1
  ads5296_snap2_adc1_e3/1 -> e3/1  "e3"
  e4_sim/1 -> ads5296_snap2_adc1_e4/1
  ads5296_snap2_adc1_e4/1 -> e4/1  "e4"
  f1_sim/1 -> ads5296_snap2_adc1_f1/1
  ads5296_snap2_adc1_f1/1 -> f1/1  "f1"
  f2_sim/1 -> ads5296_snap2_adc1_f2/1
  ads5296_snap2_adc1_f2/1 -> f2/1  "f2"
  f3_sim/1 -> ads5296_snap2_adc1_f3/1
  ads5296_snap2_adc1_f3/1 -> f3/1  "f3"
  f4_sim/1 -> ads5296_snap2_adc1_f4/1
  ads5296_snap2_adc1_f4/1 -> f4/1  "f4"
  g1_sim/1 -> ads5296_snap2_adc1_g1/1
  ads5296_snap2_adc1_g1/1 -> g1/1  "g1"
  g2_sim/1 -> ads5296_snap2_adc1_g2/1
  ads5296_snap2_adc1_g2/1 -> g2/1  "g2"
  g3_sim/1 -> ads5296_snap2_adc1_g3/1
  ads5296_snap2_adc1_g3/1 -> g3/1  "g3"
  g4_sim/1 -> ads5296_snap2_adc1_g4/1
  ads5296_snap2_adc1_g4/1 -> g4/1  "g4"
  h1_sim/1 -> ads5296_snap2_adc1_h1/1
  ads5296_snap2_adc1_h1/1 -> h1/1  "h1"
  h2_sim/1 -> ads5296_snap2_adc1_h2/1
  ads5296_snap2_adc1_h2/1 -> h2/1  "h2"
  h3_sim/1 -> ads5296_snap2_adc1_h3/1
  ads5296_snap2_adc1_h3/1 -> h3/1  "h3"
  h4_sim/1 -> ads5296_snap2_adc1_h4/1
  ads5296_snap2_adc1_h4/1 -> h4/1  "h4"
  sync/1 -> ads5296_snap2_adc1_adc_sync/1
  ads5296_snap2_adc1_adc_sync/1 -> sync_term/1
  rst/1 -> ads5296_snap2_adc1_adc_rst/1
  ads5296_snap2_adc1_adc_rst/1 -> rst_term/1
  snapshot_trig/1 -> ads5296_snap2_adc1_snapshot_ext_trigger/1
  ads5296_snap2_adc1_snapshot_ext_trigger/1 -> snapshot_trig_term/1
  sim_sync_out/1 -> ads5296_snap2_adc1_adc_sync_out/1
  ads5296_snap2_adc1_adc_sync_out/1 -> sync_out/1

== system ads5296_snap2/chan_sel ==
  sim_1 : Inport
  ads5296_snap2_chan_sel_user_data_out : xbsIndex_r4/Gateway In  gui_display_data_type=Fixed-point  arith_type=Unsigned  n_bits=32  bin_pt=0  preci_type=Single  exp_width=8  frac_width=24  rows=1  columns=1  quantization="Round  (unbiased: +/- Inf)"  overflow=Saturate  period=1  UseAsADC=off  ADCChannel='1'  interface=None  automatic_assignment=on  address_offset=hex2dec('00')  intf_name=''  intf_description=''  default_value=0  timing_constraint=None  locs_specified=off  LOCs={}  io_standard={}  inherit_from_input=off  hdl_port=on  dbl_ovrd=off  block_type=gatewayin
  convert1_1 : DataTypeConversion  OutDataTypeStr=fixdt('ufix5_En0')  LockScale=on
  convert2_1 : DataTypeConversion  OutDataTypeStr=fixdt('ufix5_En0')  ConvertRealWorld=Stored Integer (SI)  LockScale=on
  gain_1 : Gain
  io_delay : xbsIndex_r4/Delay  rst=off  infoeditControl=Selection of Reset will increase slice count due to use of real FFs and instead of SRLs  en=off  latency=0  reg_retiming=on  dbl_ovrd=off  block_type=delay
  reint1 : xbsIndex_r4/Reinterpret  force_arith_type=on  arith_type=Unsigned  force_bin_pt=on  bin_pt=0  block_type=reinterpret
  slice_reg : xbsIndex_r4/Slice  nbits=5  boolean_output=off  mode=Lower Bit Location + Width  bit1=0  base1=MSB of Input  bit0=0  base0=LSB of Input  dbl_ovrd=off  block_type=slice
  in_reg : Outport
  wires:
  ads5296_snap2_chan_sel_user_data_out/1 -> io_delay/1
  sim_1/1 -> convert1_1/1
  convert1_1/1 -> convert2_1/1
  convert2_1/1 -> gain_1/1
  gain_1/1 -> ads5296_snap2_chan_sel_user_data_out/1
  io_delay/1 -> slice_reg/1
  slice_reg/1 -> reint1/1
  reint1/1 -> in_reg/1

== system ads5296_snap2/err_cnt0 ==
  note: the two values after
      | a sync should match
  note: sample N should be 1 greater
      | than sample N-2
  note: split into even/odd cores.
      | Repeat samples. Samples separated by 2 clocks
      | should differ by 1
  note: even core
  note: sample N should be 1 greater
      | than sample N-2
  din : Inport
  AddSub : xbsIndex_r4/AddSub  mode=Addition  use_carryin=off  use_carryout=off  en=off  latency=2  precision=User Defined  arith_type=Unsigned  n_bits=10  bin_pt=0  quantization=Truncate  overflow=Wrap  use_behavioral_HDL=off  hw_selection=Fabric  pipelined=off  dbl_ovrd=off  block_type=addsub
  AddSub1 : xbsIndex_r4/AddSub  mode=Addition  use_carryin=off  use_carryout=off  en=off  latency=2  precision=User Defined  arith_type=Unsigned  n_bits=10  bin_pt=0  quantization=Truncate  overflow=Wrap  use_behavioral_HDL=off  hw_selection=Fabric  pipelined=off  dbl_ovrd=off  block_type=addsub
  Constant : xbsIndex_r4/Constant  const=1.0  gui_display_data_type=Fixed-point  arith_type=Unsigned  n_bits=1  bin_pt=0  preci_type=Single  exp_width=8  frac_width=24  explicit_period=on  period=1  equ=P=C  opselect=C  inp2=PCIN>>17  opr=+  inp1=P  carry=CIN  dbl_ovrd=off  block_type=constant
  Constant1 : xbsIndex_r4/Constant  const=1.0  gui_display_data_type=Fixed-point  arith_type=Unsigned  n_bits=1  bin_pt=0  preci_type=Single  exp_width=8  frac_width=24  explicit_period=on  period=1  equ=P=C  opselect=C  inp2=PCIN>>17  opr=+  inp1=P  carry=CIN  dbl_ovrd=off  block_type=constant
  Counter : xbsIndex_r4/Counter  cnt_type=Free Running  cnt_to=Inf  operation=Up  start_count=0  cnt_by_val=1  arith_type=Unsigned  n_bits=32  bin_pt=0  load_pin=off  rst=on  en=on  explicit_period=on  period=1  use_behavioral_HDL=off  implementation=Fabric  dbl_ovrd=off  block_type=counter
  Counter1 : xbsIndex_r4/Counter  cnt_type=Free Running  cnt_to=Inf  operation=Up  start_count=0  cnt_by_val=1  arith_type=Unsigned  n_bits=32  bin_pt=0  load_pin=off  rst=on  en=on  explicit_period=on  period=1  use_behavioral_HDL=off  implementation=Fabric  dbl_ovrd=off  block_type=counter
  Counter2 : xbsIndex_r4/Counter  cnt_type=Free Running  cnt_to=Inf  operation=Up  start_count=0  cnt_by_val=1  arith_type=Unsigned  n_bits=32  bin_pt=0  load_pin=off  rst=on  en=on  explicit_period=on  period=1  use_behavioral_HDL=off  implementation=Fabric  dbl_ovrd=off  block_type=counter
  Delay{,1..4,6} (6 alike) : xbsIndex_r4/Delay  rst=off  infoeditControl=Selection of Reset will increase slice count due to use of real FFs and instead of SRLs  en=off  latency=1  reg_retiming=off  dbl_ovrd=off  block_type=delay
  Delay5 : xbsIndex_r4/Delay  rst=off  infoeditControl=Selection of Reset will increase slice count due to use of real FFs and instead of SRLs  en=off  latency=2  reg_retiming=off  dbl_ovrd=off  block_type=delay
  Reinterpret : xbsIndex_r4/Reinterpret  force_arith_type=on  arith_type=Unsigned  force_bin_pt=on  bin_pt=0  block_type=reinterpret
  Reinterpret1 : xbsIndex_r4/Reinterpret  force_arith_type=on  arith_type=Unsigned  force_bin_pt=on  bin_pt=0  block_type=reinterpret
  Reinterpret2 : xbsIndex_r4/Reinterpret  force_arith_type=on  arith_type=Unsigned  force_bin_pt=on  bin_pt=0  block_type=reinterpret
  Relational : xbsIndex_r4/Relational  mode=a!=b  op_type=Bool  en=off  latency=1  dbl_ovrd=off  block_type=relational
  Relational1 : xbsIndex_r4/Relational  mode=a!=b  op_type=Bool  en=off  latency=1  dbl_ovrd=off  block_type=relational
  Relational2 : xbsIndex_r4/Relational  mode=a!=b  op_type=Bool  en=on  latency=1  dbl_ovrd=off  block_type=relational
  interleave_err_cnt : Subsystem  Tag=xps:sw_reg  AncestorBlock=xps_library/Memory/software_register  mask(swreg){io_dir=To Processor, io_delay=0, init_val=0, sample_period=1, names=reg, bitwidths=32, bin_pts=0, arith_types=0, sim_port=on, show_format=on}
      mask prompts: io_dir "I/O direction"; io_delay "I/O delay"; init_val "Initial Value"; sample_period "Sample period"; names "Bitfield names [msb...lsb]"; bitwidths "Bitfield widths"; bin_pts "Bitfield binary pts"; arith_types "Bitfield types, ufix=0, fix=1, bool=2"; sim_port "Provide sim input/output?"; show_format "Print format string?"
      mask help: A 32-bit software-accessible register. Can be divided into bitfields of varying widths and types using the fields in the block mask.
      mask init:
      | swreg_init(gcb)
      settings: AttributesFormatString=1output:uf32.0 = 32 bits
      mask TypeOptions io_dir: To Processor | From Processor
      mask Callback io_dir:
      | mask_enables = get_param(gcb, 'MaskEnables');
      | mask_names = get_param(gcb, 'MaskNames');
      | if strcmp(get_param(gcb, 'io_dir'), 'To Processor'),
      |     mask_enables{ismember(mask_names, 'sample_period')} = 'off';
      | else
      |     mask_enables{ismember(mask_names, 'sample_period')} = 'on';
      | end
      | set_param(gcb, 'MaskEnables', mask_enables);
      mask DialogControl ParameterTabVar0 Prompt: Setup
  ramp_err_cnt0 : Subsystem  Tag=xps:sw_reg  AncestorBlock=xps_library/Memory/software_register  mask(swreg){io_dir=To Processor, io_delay=0, init_val=0, sample_period=1, names=reg, bitwidths=32, bin_pts=0, arith_types=0, sim_port=on, show_format=on}
      mask prompts: io_dir "I/O direction"; io_delay "I/O delay"; init_val "Initial Value"; sample_period "Sample period"; names "Bitfield names [msb...lsb]"; bitwidths "Bitfield widths"; bin_pts "Bitfield binary pts"; arith_types "Bitfield types, ufix=0, fix=1, bool=2"; sim_port "Provide sim input/output?"; show_format "Print format string?"
      mask help: A 32-bit software-accessible register. Can be divided into bitfields of varying widths and types using the fields in the block mask.
      mask init:
      | swreg_init(gcb)
      settings: AttributesFormatString=1output:uf32.0 = 32 bits
      mask TypeOptions io_dir: To Processor | From Processor
      mask Callback io_dir:
      | mask_enables = get_param(gcb, 'MaskEnables');
      | mask_names = get_param(gcb, 'MaskNames');
      | if strcmp(get_param(gcb, 'io_dir'), 'To Processor'),
      |     mask_enables{ismember(mask_names, 'sample_period')} = 'off';
      | else
      |     mask_enables{ismember(mask_names, 'sample_period')} = 'on';
      | end
      | set_param(gcb, 'MaskEnables', mask_enables);
      mask DialogControl ParameterTabVar0 Prompt: Setup
  ramp_err_cnt1 : Subsystem  Tag=xps:sw_reg  AncestorBlock=xps_library/Memory/software_register  mask(swreg){io_dir=To Processor, io_delay=0, init_val=0, sample_period=1, names=reg, bitwidths=32, bin_pts=0, arith_types=0, sim_port=on, show_format=on}
      mask prompts: io_dir "I/O direction"; io_delay "I/O delay"; init_val "Initial Value"; sample_period "Sample period"; names "Bitfield names [msb...lsb]"; bitwidths "Bitfield widths"; bin_pts "Bitfield binary pts"; arith_types "Bitfield types, ufix=0, fix=1, bool=2"; sim_port "Provide sim input/output?"; show_format "Print format string?"
      mask help: A 32-bit software-accessible register. Can be divided into bitfields of varying widths and types using the fields in the block mask.
      mask init:
      | swreg_init(gcb)
      settings: AttributesFormatString=1output:uf32.0 = 32 bits
      mask TypeOptions io_dir: To Processor | From Processor
      mask Callback io_dir:
      | mask_enables = get_param(gcb, 'MaskEnables');
      | mask_names = get_param(gcb, 'MaskNames');
      | if strcmp(get_param(gcb, 'io_dir'), 'To Processor'),
      |     mask_enables{ismember(mask_names, 'sample_period')} = 'off';
      | else
      |     mask_enables{ismember(mask_names, 'sample_period')} = 'on';
      | end
      | set_param(gcb, 'MaskEnables', mask_enables);
      mask DialogControl ParameterTabVar0 Prompt: Setup
  square_transposer : Subsystem  AncestorBlock=casper_library_reorder/square_transposer  mask(square_transposer){n_inputs=1, async=off}
      mask prompts: n_inputs "Number of inputs (2^?):"; async "Aynchronus operation"
      mask init:
      | square_transposer_init(gcb,...
      |     'n_inputs', n_inputs, ...
      |     'async', async);
      settings: AttributesFormatString=n_inputs=1
      mask Help: eval('xlWeb(''http://casper.berkeley.edu/wiki/Square_transposer'')')
  dout : Outport
  wires:
  din/1 -> Reinterpret2/1, dout/1
  Reinterpret/1 -> Relational/1, AddSub/1
  Constant/1 -> AddSub/2
  AddSub/1 -> Relational/2
  Counter/1 -> ramp_err_cnt0/1(out_reg)
  Relational/1 -> Counter/2
  [err_cnt_rst] -> Delay/1
  Delay/1 -> Counter/1
  [sync] -> Delay2/1
  square_transposer/2(out0) -> Reinterpret/1
  Delay1/1 -> Counter1/1
  [err_cnt_rst] -> Delay1/1
  Relational1/1 -> Counter1/2
  Counter1/1 -> ramp_err_cnt1/1(out_reg)
  AddSub1/1 -> Relational1/2
  Constant1/1 -> AddSub1/2
  Reinterpret1/1 -> AddSub1/1, Relational1/1
  square_transposer/3(out1) -> Reinterpret1/1
  Delay2/1 -> square_transposer/1(sync)
  Delay3/1 -> square_transposer/3(in1), square_transposer/2(in0)
  Delay4/1 -> Relational2/2
  Delay5/1 -> Relational2/3
  Reinterpret2/1 -> Delay4/1, Relational2/1, Delay3/1
  Counter2/1 -> interleave_err_cnt/1(out_reg)
  [err_cnt_rst] -> Delay6/1
  Delay6/1 -> Counter2/1
  Relational2/1 -> Counter2/2
  [sync] -> Delay5/1
